simulink subsystem "Dyn_Params"  (R2024b)
settings: Solver=VariableStepAuto  StartTime=0.0  StopTime=10.0  RelTol=1e-3
undefined symbols (not defined in the file): SimPar
settings Model: Creator=bmsimmon  LastModifiedBy=macheson
settings RTWCC: GPUComputeCapability=3.5

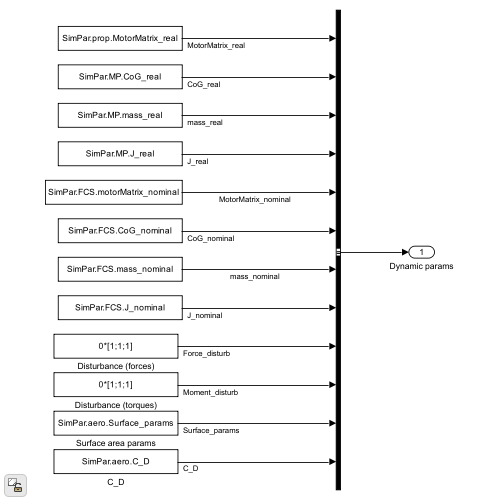
[thumbnail: Simulink's stored preview of the top-level diagram]
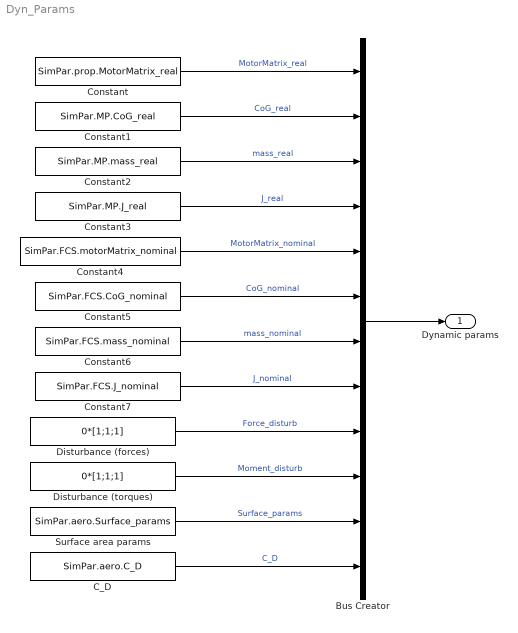
== system Dyn_Params ==
  Bus Creator : BusCreator  Inputs=12
  C_D : Constant  Value=SimPar.aero.C_D
  Constant : Constant  Value=SimPar.prop.MotorMatrix_real
  Constant1 : Constant  Value=SimPar.MP.CoG_real
  Constant2 : Constant  Value=SimPar.MP.mass_real
  Constant3 : Constant  Value=SimPar.MP.J_real
  Constant4 : Constant  Value=SimPar.FCS.motorMatrix_nominal
  Constant5 : Constant  Value=SimPar.FCS.CoG_nominal
  Constant6 : Constant  Value=SimPar.FCS.mass_nominal
  Constant7 : Constant  Value=SimPar.FCS.J_nominal
  Disturbance (forces) : Constant  Value=0*[1;1;1]
  Disturbance (torques) : Constant  Value=0*[1;1;1]
  Surface area params : Constant  Value=SimPar.aero.Surface_params
  Dynamic params : Outport  VectorParamsAs1DForOutWhenUnconnected=off
  wires:
  Bus Creator/1 -> Dynamic params/1
  Constant/1 -> Bus Creator/1  "MotorMatrix_real"
  Constant1/1 -> Bus Creator/2  "CoG_real"
  Constant3/1 -> Bus Creator/4  "J_real"
  Surface area params/1 -> Bus Creator/11  "Surface_params"
  Disturbance (forces)/1 -> Bus Creator/9  "Force_disturb"
  Constant4/1 -> Bus Creator/5  "MotorMatrix_nominal"
  Constant5/1 -> Bus Creator/6  "CoG_nominal"
  Constant6/1 -> Bus Creator/7  "mass_nominal"
  Constant7/1 -> Bus Creator/8  "J_nominal"
  Disturbance (torques)/1 -> Bus Creator/10  "Moment_disturb"
  Constant2/1 -> Bus Creator/3  "mass_real"
  C_D/1 -> Bus Creator/12  "C_D"
